simulink model "wbme_example_sim"  (R2018b)
settings: Solver=ode45  StartTime=0.0  StopTime=10  FixedStep=sample_time  RelTol=1e-3
values from neighbouring files (symbols this model uses):
  imu_acc_bias = (rand(num_IMUs,1) - 0.5) * 0    [wbme_example_init_sim.m]
  imu_gyro_bias = (rand(num_IMUs,1) - 0.5) * 0    [wbme_example_init_sim.m]
  Phi_az_sim = WBME.eta_scale * Phi_az_sim    [wbme_example_init_sim.m]
  Phi_roll_sim = WBME.eta_scale * Phi_roll_sim    [wbme_example_init_sim.m]
  Phi_s_sim = WBME.eta_scale * Phi_s_sim    [wbme_example_init_sim.m]
  structure = structureCreate('structure_params_Funray_soft')    [wbme_example_init_sim.m]
  structure_red = structureGetReduced(structure,num_modes)    [wbme_example_init_sim.m]
undefined symbols (not defined in the file or in its folder): structureGetNodeCg, structureGetNodeMass, structureGetTotalInertia, structureGetTotalMass, WBME_notune
libraries: simulink x3, filters_lib x1, flexibleBody_lib x1, wbme_lib x1
settings Model: Creator=milic  LastModifiedBy=yannic

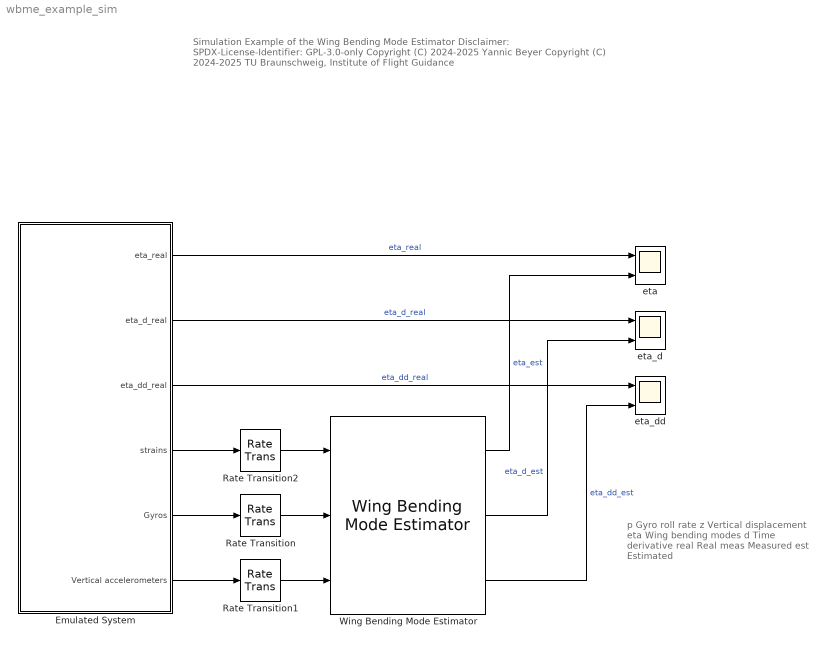
== system wbme_example_sim ==
  note: p
      | Gyro roll rate
      |
      | z
      | Vertical displacement
      |
      | eta
      | Wing bending modes
      |
      | d
      | Time derivative
      |
      | real
      | Real
      |
      | meas
      | Measured
      |
      | est
      | Estimated
  note: Simulation Example of the Wing Bending Mode Estimator
      |
      | Disclaimer:
      | SPDX-License-Identifier: GPL-3.0-only
      |
      | Copyright (C) 2024-2025 Yannic Beyer
      | Copyright (C) 2024-2025 TU Braunschweig, Institute of Flight Guidance
  Emulated System : Subsystem
  Rate Transition : RateTransition
  Rate Transition1 : RateTransition
  Rate Transition2 : RateTransition
  Wing Bending Mode Estimator : wbme_lib/Wing Bending Mode Estimator  wbmo=WBME  wbmo_notune=WBME_notune
  eta : Scope  NumInputPorts=2
  eta_d : Scope  NumInputPorts=2
  eta_dd : Scope  NumInputPorts=2
  wires:
  Wing Bending Mode Estimator/3 -> eta_dd/2  "eta_dd_est"
  Wing Bending Mode Estimator/1 -> eta/2  "eta_est"
  Wing Bending Mode Estimator/2 -> eta_d/2  "eta_d_est"
  Emulated System/1(eta_real) -> eta/1  "eta_real"
  Emulated System/5(Gyros) -> Rate Transition/1
  Emulated System/2(eta_d_real) -> eta_d/1  "eta_d_real"
  Emulated System/6(Vertical accelerometers) -> Rate Transition1/1
  Emulated System/3(eta_dd_real) -> eta_dd/1  "eta_dd_real"
  Rate Transition/1 -> Wing Bending Mode Estimator/2
  Rate Transition1/1 -> Wing Bending Mode Estimator/3
  Emulated System/4(strains) -> Rate Transition2/1
  Rate Transition2/1 -> Wing Bending Mode Estimator/1

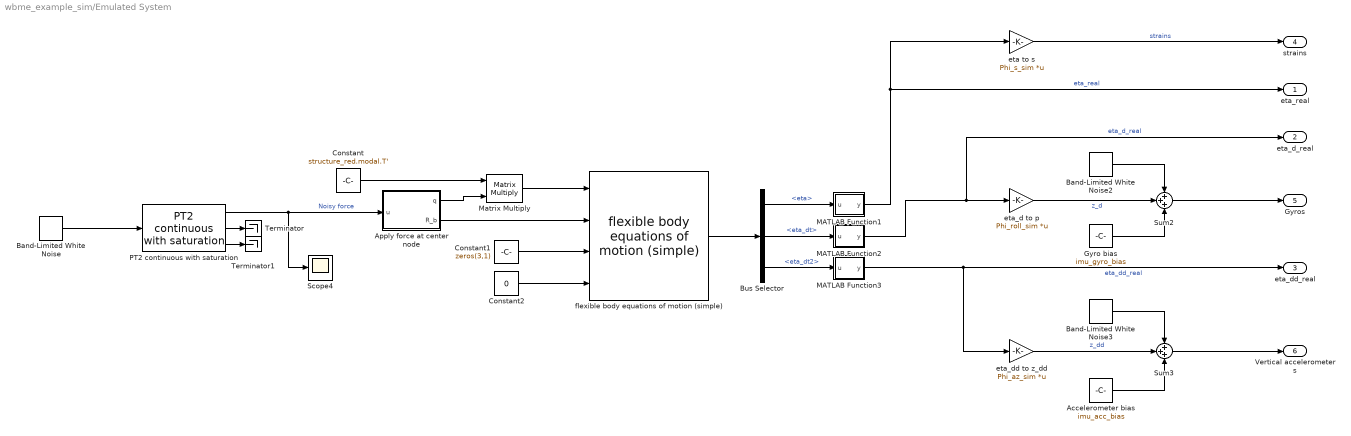
== system wbme_example_sim/Emulated System ==
  Accelerometer bias : Constant  Value=imu_acc_bias
  Apply force at center node : MATLAB Function  TreatAsAtomicUnit=on
  Band-Limited White Noise : simulink/Sources/Band-Limited White Noise  Cov=2  Ts=WBME_notune.sample_time  seed=[23341]
  Band-Limited White Noise2 : simulink/Sources/Band-Limited White Noise  Cov=0  Ts=WBME_notune.sample_time  seed=1:size(Phi_az_sim,1)
  Band-Limited White Noise3 : simulink/Sources/Band-Limited White Noise  Cov=0  Ts=WBME_notune.sample_time  seed=1:size(Phi_az_sim,1)
  Bus Selector : BusSelector  OutputSignals=eta,eta_dt,eta_dt2
  Constant : Constant  Value=structure_red.modal.T'
  Constant1 : Constant  Value=zeros(3,1)
  Constant2 : Constant  Value=0
  Gyro bias : Constant  Value=imu_gyro_bias
  MATLAB Function1 : MATLAB Function  TreatAsAtomicUnit=on
  MATLAB Function2 : MATLAB Function  TreatAsAtomicUnit=on
  MATLAB Function3 : MATLAB Function  TreatAsAtomicUnit=on
  Matrix Multiply : Product  Multiplication=Matrix(*)
  PT2 continuous with saturation : filters_lib/PT2 continuous with saturation  omega=150  d=0.7  x_dt2_max=inf  x_dt2_min=-inf  x_dt_max=inf  x_dt_min=-inf  x_max=inf  x_min=-inf  x_init=0  x_dt_init=0
      settings: SourceProductName=LADAC
  Scope4 : Scope
  Sum2 : Sum  Inputs=+++
  Sum3 : Sum  Inputs=+++
  Terminator : Terminator
  Terminator1 : Terminator
  eta to s : Gain  Gain=Phi_s_sim  Multiplication=Matrix(K*u)
  eta_d to p : Gain  Gain=Phi_roll_sim  Multiplication=Matrix(K*u)
  eta_dd to z_dd : Gain  Gain=Phi_az_sim  Multiplication=Matrix(K*u)
  flexible body equations of motion (simple) : flexibleBody_lib/flexible body equations of motion (simple)  structure_red=structure_red  m=structureGetTotalMass(structure)  I_b=structureGetTotalInertia(structure)  m_nodes=structureGetNodeMass(structure,1:length(structure.xyz))  cg_nodes=structureGetNodeCg(structure,1:length(structure.xyz))  structure_vel_0=zeros(size(structure_red.K,2)-6,1)  structure_pos_0=zeros(size(structure_red.K,2)-6,1)
      settings: SourceProductName=LADAC
  eta_real : Outport
  eta_d_real : Outport  Port=2
  eta_dd_real : Outport  Port=3
  strains : Outport  Port=4
  Gyros : Outport  Port=5
  Vertical accelerometers : Outport  Port=6
  wires:
  Constant/1 -> Matrix Multiply/1
  eta_dd to z_dd/1 -> Sum3/2  "z_dd"
  PT2 continuous with saturation/3 -> Terminator1/1
  Matrix Multiply/1 -> flexible body equations of motion (simple)/1
  Accelerometer bias/1 -> Sum3/3
  MATLAB Function2/1(y) -> eta_d to p/1, eta_d_real/1  "eta_d_real"
  Sum2/1 -> Gyros/1
  Band-Limited White Noise3/1 -> Sum3/1
  MATLAB Function1/1(y) -> eta_real/1, eta to s/1  "eta_real"
  MATLAB Function3/1(y) -> eta_dd_real/1, eta_dd to z_dd/1  "eta_dd_real"
  Bus Selector/2 -> MATLAB Function2/1(u)  "<eta_dt>"
  Constant1/1 -> flexible body equations of motion (simple)/3
  Sum3/1 -> Vertical accelerometers/1
  PT2 continuous with saturation/2 -> Terminator/1
  Apply force at center node/2(R_b) -> flexible body equations of motion (simple)/2
  Constant2/1 -> flexible body equations of motion (simple)/4
  flexible body equations of motion (simple)/1 -> Bus Selector/1
  PT2 continuous with saturation/1 -> Scope4/1, Apply force at center node/1(u)  "Noisy force"
  Band-Limited White Noise/1 -> PT2 continuous with saturation/1
  eta_d to p/1 -> Sum2/2  "z_d"
  Apply force at center node/1(q) -> Matrix Multiply/2
  Bus Selector/1 -> MATLAB Function1/1(u)  "<eta>"
  Bus Selector/3 -> MATLAB Function3/1(u)  "<eta_dt2>"
  Band-Limited White Noise2/1 -> Sum2/1
  Gyro bias/1 -> Sum2/3
  eta to s/1 -> strains/1  "strains"

== matlab function wbme_example_sim/Emulated System/Apply force at center node ==
  data: u input; q output; R_b output; num_nodes parameter
function [q,R_b] = fcn(u,num_nodes)
q = zeros(6*num_nodes,1);
q((num_nodes/2-0.5)*6+3) = u;
R_b = zeros(3,1);
R_b(3) = u;
end

== matlab function wbme_example_sim/Emulated System/MATLAB Function1 ==
  data: u input; y output
function y = fcn(u)
y = u(7:end);
end

== matlab function wbme_example_sim/Emulated System/MATLAB Function2 ==
  data: u input; y output
function y = fcn(u)
y = u(7:end);
end

== matlab function wbme_example_sim/Emulated System/MATLAB Function3 ==
  data: u input; y output
function y = fcn(u)
y = u(7:end);
end
